simulink model "CubliSenseToolSimOLD"  (R2015a)
settings: Solver=ode45  StartTime=0.0  StopTime=5  RelTol=1e-3
values from neighbouring files (symbols this model uses):
  B_f = 6.08e-3    (= 0.00608)    [CubliSenseTool.m]
  g = 9.82    [CubliSenseTool.m]
  J_f = (2.8e-3)    (= 0.0028)    [CubliSenseTool.m]
  J_w = 0.601e-3    (= 0.000601)    [CubliSenseTool.m]
  l_f = 0.076    [CubliSenseTool.m]
  l_w = 0.093    [CubliSenseTool.m]
  m_f = 0.354    [CubliSenseTool.m]
  m_w = 0.222    [CubliSenseTool.m]
settings Model: Creator=vniel  LastModifiedBy=USUARIO
settings DataIOCC: Refine=25

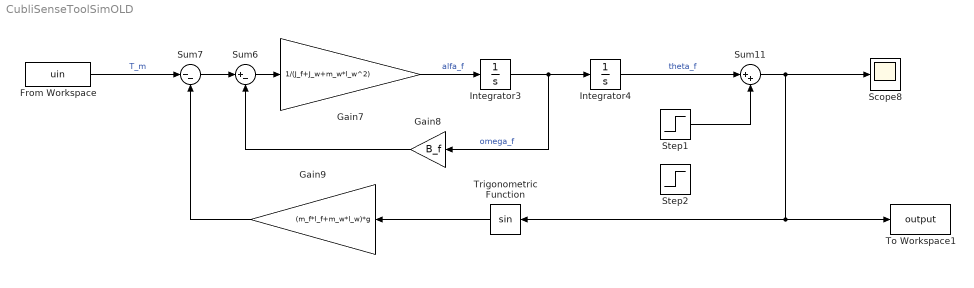
== system CubliSenseToolSimOLD ==
  From Workspace : FromWorkspace  VariableName=uin  SampleTime=0.01
  Gain7 : Gain  Gain=1/(J_f+J_w+m_w*l_w^2)
  Gain8 : Gain  Gain=B_f
  Gain9 : Gain  Gain=(m_f*l_f+m_w*l_w)*g
  Integrator3 : Integrator
  Integrator4 : Integrator
  Scope8 : Scope
      settings: TimeRange=auto  LimitDataPoints=on  MaxDataPoints=5000  SaveToWorkspace=off  SaveName=ScopeData6  YMin=-10  YMax=10  SampleTime=-1
  Step1 : Step  Time=0  After=0.1286  SampleTime=0
  Step2 : Step  Time=0  After=-0.09023  SampleTime=0
  Sum11 : Sum  Inputs=|++
  Sum6 : Sum  Inputs=|+-
  Sum7 : Sum  Inputs=|--
  To Workspace1 : ToWorkspace  VariableName=output  SampleTime=0.0025
      settings: MaxDataPoints=2000
  Trigonometric Function : Trigonometry
  wires:
  Gain7/1 -> Integrator3/1  "alfa_f"
  Integrator3/1 -> Gain8/1, Integrator4/1  "omega_f"
  Sum6/1 -> Gain7/1
  Sum7/1 -> Sum6/1
  Gain8/1 -> Sum6/2
  Gain9/1 -> Sum7/2
  Integrator4/1 -> Sum11/1  "theta_f"
  Trigonometric Function/1 -> Gain9/1
  From Workspace/1 -> Sum7/1  "T_m"
  Sum11/1 -> Trigonometric Function/1, To Workspace1/1, Scope8/1
  Step1/1 -> Sum11/2
